simulink model "SLDCMotor_FPvsPM"  (R2018b)
settings: Solver=ode15s  StartTime=0.0  StopTime=5  RelTol=1e-3  EnableMultiTasking=on
PreLoadFcn:
  | J=0.01;
  | Kf=0.1;
  | K=0.01;
  | R=1;
  | L=0.5;
libraries: fl_lib x15, nesl_utility x6, elec_lib x1
settings Model: Creator=cosorio  LastModifiedBy=jlesage
settings DataIOCC: LimitDataPoints=on  SaveFormat=Array  SignalLoggingSaveFormat=ModelDataLogs  SaveTime=off
settings OptimizationCC: ExpressionDepthLimit=2147483647  LifeSpan=inf
settings DebuggingCC: UnderspecifiedInitializationDetection=Classic  MergeDetectMultiDrivingBlocksExec=none  FcnCallInpInsideContextMsg=warning  AllowSymbolicDim=off  StateNameClashWarn=warning  SFUnexpectedBacktrackingDiag=warning  SFNoUnconditionalDefaultTransitionDiag=warning  SFExecutionAtInitializationDiag=none
settings HardwareCC: ProdBitPerPointer=32  ProdBitPerSizeT=32  ProdBitPerPtrDiffT=32  ProdLargestAtomicFloat=None  ProdIntDivRoundTo=Undefined  ProdEndianess=Unspecified  ProdWordSize=32  ProdHWDeviceType=32-bit Generic
settings ModelReferenceCC: PropagateSignalLabelsOutOfModel=off
settings SFSimCC: SimUseLocalCustomCode=off
settings RTWCC: RTWUseLocalCustomCode=off
settings CodeAppCC: StateflowObjectComments=on
settings GRTTargetCC: TargetLangStandard=C89/C90 (ANSI)  GeneratePreprocessorConditionals=Disable all  CombineOutputUpdateFcns=off  GRTInterface=on
settings ConfigComp: CovMetricSettings=dw  CovHtmlReporting=on  CovSaveCumulativeToWorkspaceVar=on  CovSaveSingleToWorkspaceVar=on  CovExternalEMLEnable=off  CovSFcnEnable=off
settings SimscapeCC: SimscapeNormalizeSystem=off

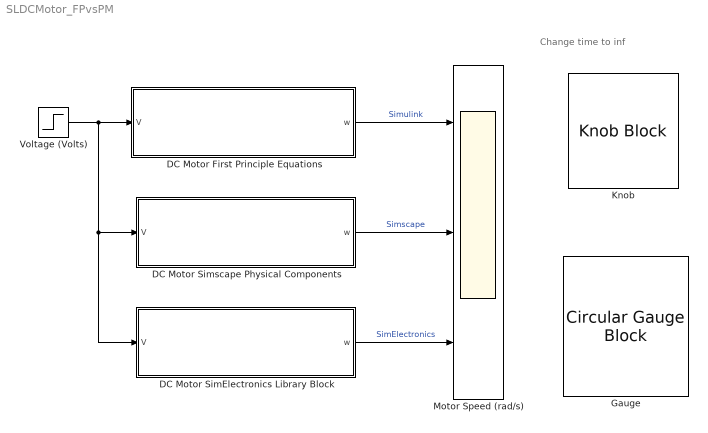
== system SLDCMotor_FPvsPM ==
  note: Change time to inf
  DC Motor First Principle Equations : Subsystem
  DC Motor SimElectronics Library Block : Subsystem
  DC Motor Simscape Physical Components : Subsystem
  Gauge : CircularGaugeBlock  WebBlockId=66  ScaleMax=1
  Knob : KnobBlock  WebBlockId=65  ScaleMax=5
  Motor Speed (rad/s) : Scope  NumInputPorts=3
  Voltage (Volts) : Step  After=0.9655958811442057  SampleTime=0
  wires:
  Voltage (Volts)/1 -> DC Motor First Principle Equations/1(V), DC Motor Simscape Physical Components/1(V), DC Motor SimElectronics Library Block/1(V)
  DC Motor First Principle Equations/1(w) -> Motor Speed (rad/s)/1  "Simulink"
  DC Motor Simscape Physical Components/1(w) -> Motor Speed (rad/s)/2  "Simscape"
  DC Motor SimElectronics Library Block/1(w) -> Motor Speed (rad/s)/3  "SimElectronics"

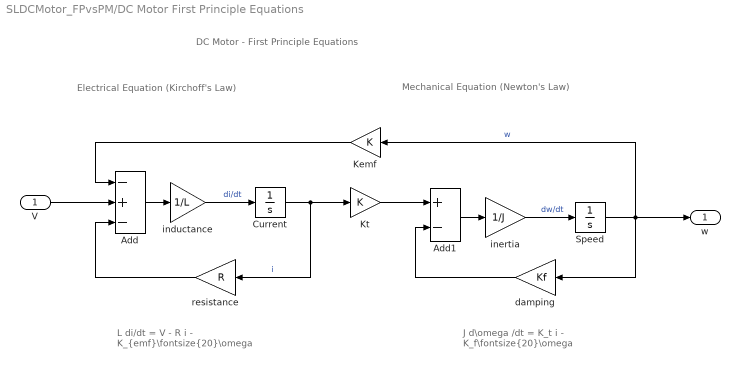
== system SLDCMotor_FPvsPM/DC Motor First Principle Equations ==
  note: Mechanical Equation
      |                 (Newton's Law)
  note: Electrical Equation
      |                 (Kirchoff's Law)
  note: L di/dt = V - R i - K_{emf}\fontsize{20}\omega
  note: J d\omega /dt = K_t i - K_f\fontsize{20}\omega
  note: DC Motor - First Principle Equations
  V : Inport
  Add : Sum  Inputs=-+-
  Add1 : Sum  Inputs=+-
  Current : Integrator
  Kemf : Gain  Gain=K
  Kt : Gain  Gain=K
  Speed : Integrator
  damping : Gain  Gain=Kf
  inductance : Gain  Gain=1/L
  inertia : Gain  Gain=1/J
  resistance : Gain  Gain=R
  w : Outport
  wires:
  V/1 -> Add/2
  inertia/1 -> Speed/1  "dw/dt"
  damping/1 -> Add1/2
  Kt/1 -> Add1/1
  inductance/1 -> Current/1  "di/dt"
  Speed/1 -> w/1, damping/1, Kemf/1  "w"
  Add1/1 -> inertia/1
  Current/1 -> Kt/1, resistance/1  "i"
  Add/1 -> inductance/1
  resistance/1 -> Add/3
  Kemf/1 -> Add/1

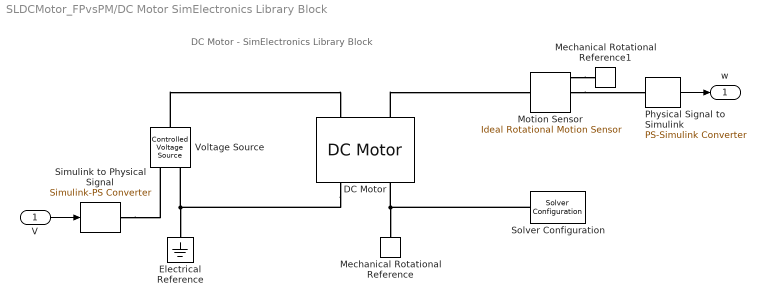
== system SLDCMotor_FPvsPM/DC Motor SimElectronics Library Block ==
  note: DC Motor - SimElectronics Library Block
  V : Inport
  DC Motor : elec_lib/Actuators & Drivers/Rotational Actuators/DC Motor  parameterization=1  Ra=R Ohm  La=L H  emf_or_torque=2  Kv=7.2e-05 V/rpm  Ki=K N*m/A  T_stall=2.4e-04 N*m  w_max=1.91e+04 rpm  w_rated=1.5e+04 rpm  P_rated=0.08 W  V_rated=1.5 V  J=J kg*m^2  lam_param=1  lam=Kf N*m/(rad/s)  i_noload=0 A  V_i_noload=1.5 V  speed0=0 rpm  alpha=0.00393 1/K  Tmeas=25 C  thermal_mass=100 J/K  initial_temperature=25 C
  Electrical Reference : fl_lib/Electrical/Electrical Elements/Electrical Reference
  Mechanical Rotational Reference : fl_lib/Mechanical/Rotational Elements/Mechanical Rotational Reference
  Mechanical Rotational Reference1 : fl_lib/Mechanical/Rotational Elements/Mechanical Rotational Reference
  Motion Sensor : fl_lib/Mechanical/Mechanical Sensors/Ideal Rotational Motion Sensor  offset=0 rad
  Physical Signal to Simulink : nesl_utility/PS-Simulink Converter  PhysicalDomain=network_engine_domain  SubClassName=ps_output  LeftPortType=input  RightPortType=output  PseudoPeriodic=off  Frequencies=[]  Unit=rad/s  AffineConversion=off
  Simulink to Physical Signal : nesl_utility/Simulink-PS Converter  PhysicalDomain=network_engine_domain  SubClassName=ps_input  LeftPortType=input  RightPortType=output  PseudoPeriodic=off  Frequencies=[]  NoiseDistribution=none  NoiseParameters=[]  Unit=V  AffineConversion=off  FilteringAndDerivatives=zero  SimscapeFilterOrder=1  InputFilterTimeConstant=.001  UdotUserProvided=0
  Solver Configuration : nesl_utility/Solver Configuration  PhysicalDomain=network_engine_domain  SubClassName=solver  LeftPortType=input  RightPortType=generic  Tones=[]  Harmonics=[]  SimulateNoise=off  Profile=off  UseLocalSampling=off  EnableSwitchedLinearOptims=on  FrequencyDomain=off  UseCCode=off  RelTol=0.001  AbsTol=1e-06  MinStep=1e-09  ToWorkspace=off  RevertToSquareIcSolve=off  NumHomotopyIterations=100  PhasorMode=off  PhasorModeNumHarmonics=1  DoDC=off  ResidualTolerance=1e-9  UseLocalSolver=off  LocalSolverChoice=NE_BACKWARD_EULER_ADVANCER  LocalSolverSampleTime=.001  DoFixedCost=off  MaxNonlinIter=12  MaxModeIter=2  LinearAlgebra=Sparse  EquationFormulation=NE_TIME_EF  DelaysMemoryBudget=1024  AutomaticFiltering=on  FilteringTimeConstant=0.001  PartitionStorageMethod=AS_NEEDED  PartitionMemoryBudget=1024
  Voltage Source : fl_lib/Electrical/Electrical Sources/Controlled Voltage Source
  w : Outport
  wires:
  V/1 -> Simulink to Physical Signal/1
  Physical Signal to Simulink/1 -> w/1
  connections:
  Simulink to Physical Signal/RConn1 -- Voltage Source/RConn1
  Voltage Source/LConn1 -- DC Motor/LConn1
  DC Motor/RConn1 -- Voltage Source/RConn2 -- Electrical Reference/LConn1
  Motion Sensor/RConn2 -- Physical Signal to Simulink/LConn1
  DC Motor/LConn2 -- Motion Sensor/LConn1
  Solver Configuration/RConn1 -- DC Motor/RConn2 -- Mechanical Rotational Reference/LConn1
  Motion Sensor/RConn1 -- Mechanical Rotational Reference1/LConn1

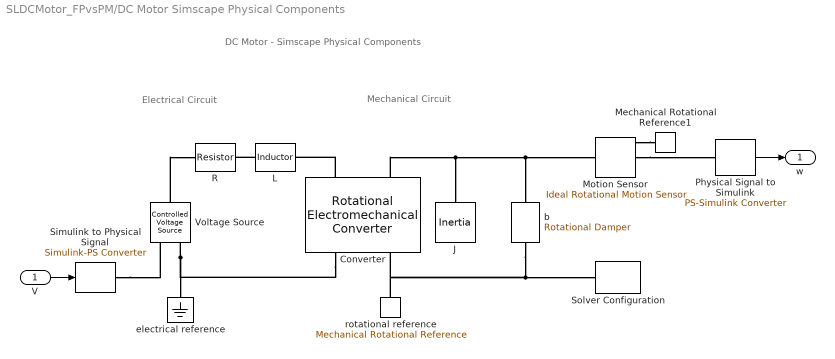
== system SLDCMotor_FPvsPM/DC Motor Simscape Physical Components ==
  note: Mechanical Circuit
  note: Electrical Circuit
  note: DC Motor - Simscape Physical Components
  V : Inport
  Converter : fl_lib/Electrical/Electrical Elements/Rotational Electromechanical Converter  K=K V/(rad/s)  i_specify=off  i_priority=High  i=0 A  i_nominal_specify=off  i_nominal_unit=A  i_nominal_value=1  v_specify=off  v_priority=High  v=0 V  v_nominal_specify=off  v_nominal_unit=V  v_nominal_value=1  t_specify=off  t_priority=High  t=0 N*m  t_nominal_specify=off  t_nominal_unit=N*m  t_nominal_value=1  w_specify=off  w_priority=High  w=0 rad/s  w_nominal_specify=off  w_nominal_unit=rad/s  w_nominal_value=1
      settings: SourceProductName=Simscape
  J : fl_lib/Mechanical/Rotational Elements/Inertia  inertia=J kg*m^2  w_specify=on  w_priority=High  w=0 rad/s  w_nominal_specify=off  w_nominal_unit=rad/s  w_nominal_value=1  t_specify=off  t_priority=High  t=0 N*m  t_nominal_specify=off  t_nominal_unit=N*m  t_nominal_value=1
  L : fl_lib/Electrical/Electrical Elements/Inductor  l=L H  r=0 Ohm  g=1e-09 1/Ohm  i_specify=off  i_priority=High  i=0 A  i_nominal_specify=off  i_nominal_unit=A  i_nominal_value=1  v_specify=off  v_priority=High  v=0 V  v_nominal_specify=off  v_nominal_unit=V  v_nominal_value=1  i_L_specify=on  i_L_priority=High  i_L=0 A  i_L_nominal_specify=off  i_L_nominal_unit=A  i_L_nominal_value=1
  Mechanical Rotational Reference1 : fl_lib/Mechanical/Rotational Elements/Mechanical Rotational Reference
  Motion Sensor : fl_lib/Mechanical/Mechanical Sensors/Ideal Rotational Motion Sensor  offset=0 rad
  Physical Signal to Simulink : nesl_utility/PS-Simulink Converter  PhysicalDomain=network_engine_domain  SubClassName=ps_output  LeftPortType=input  RightPortType=output  PseudoPeriodic=off  Frequencies=[]  Unit=rad/s  AffineConversion=off
  R : fl_lib/Electrical/Electrical Elements/Resistor  Tag=Factory Generic  R=R Ohm  i_specify=off  i_priority=High  i=0 A  i_nominal_specify=off  i_nominal_unit=A  i_nominal_value=1  v_specify=off  v_priority=High  v=0 V  v_nominal_specify=off  v_nominal_unit=V  v_nominal_value=1
  Simulink to Physical Signal : nesl_utility/Simulink-PS Converter  PhysicalDomain=network_engine_domain  SubClassName=ps_input  LeftPortType=input  RightPortType=output  PseudoPeriodic=off  Frequencies=[]  NoiseDistribution=none  NoiseParameters=[]  Unit=V  AffineConversion=off  FilteringAndDerivatives=zero  SimscapeFilterOrder=1  InputFilterTimeConstant=.001  UdotUserProvided=0
  Solver Configuration : nesl_utility/Solver Configuration  PhysicalDomain=network_engine_domain  SubClassName=solver  LeftPortType=input  RightPortType=generic  Tones=[]  Harmonics=[]  SimulateNoise=off  Profile=off  UseLocalSampling=off  EnableSwitchedLinearOptims=on  FrequencyDomain=off  UseCCode=off  RelTol=0.001  AbsTol=1e-06  MinStep=1e-09  ToWorkspace=off  RevertToSquareIcSolve=off  NumHomotopyIterations=100  PhasorMode=off  PhasorModeNumHarmonics=1  DoDC=off  ResidualTolerance=1e-9  UseLocalSolver=off  LocalSolverChoice=NE_BACKWARD_EULER_ADVANCER  LocalSolverSampleTime=.001  DoFixedCost=off  MaxNonlinIter=12  MaxModeIter=2  LinearAlgebra=Sparse  EquationFormulation=NE_TIME_EF  DelaysMemoryBudget=1024  AutomaticFiltering=on  FilteringTimeConstant=0.001  PartitionStorageMethod=AS_NEEDED  PartitionMemoryBudget=1024
  Voltage Source : fl_lib/Electrical/Electrical Sources/Controlled Voltage Source
  b : fl_lib/Mechanical/Rotational Elements/Rotational Damper  D=Kf N*m/(rad/s)  w_specify=off  w_priority=High  w=0 rad/s  w_nominal_specify=off  w_nominal_unit=rad/s  w_nominal_value=1  t_specify=off  t_priority=High  t=0 N*m  t_nominal_specify=off  t_nominal_unit=N*m  t_nominal_value=1
  electrical reference : fl_lib/Electrical/Electrical Elements/Electrical Reference
  rotational reference : fl_lib/Mechanical/Rotational Elements/Mechanical Rotational Reference
  w : Outport
  wires:
  V/1 -> Simulink to Physical Signal/1
  Physical Signal to Simulink/1 -> w/1
  connections:
  Simulink to Physical Signal/RConn1 -- Voltage Source/RConn1
  Voltage Source/LConn1 -- R/LConn1
  Voltage Source/RConn2 -- electrical reference/LConn1 -- Converter/RConn1
  rotational reference/LConn1 -- Converter/RConn2 -- Solver Configuration/RConn1 -- b/RConn1
  Converter/LConn1 -- L/RConn1
  L/LConn1 -- R/RConn1
  Converter/LConn2 -- Motion Sensor/LConn1 -- b/LConn1 -- J/LConn1
  Motion Sensor/RConn2 -- Physical Signal to Simulink/LConn1
  Motion Sensor/RConn1 -- Mechanical Rotational Reference1/LConn1
